simulink model "DynamicSimulator"  (R2016b)
settings: Solver=VariableStepAuto  StartTime=0.0  StopTime=inf  RelTol=1e-3
settings Model: Creator=Zikinkeria  LastModifiedBy=rcooper

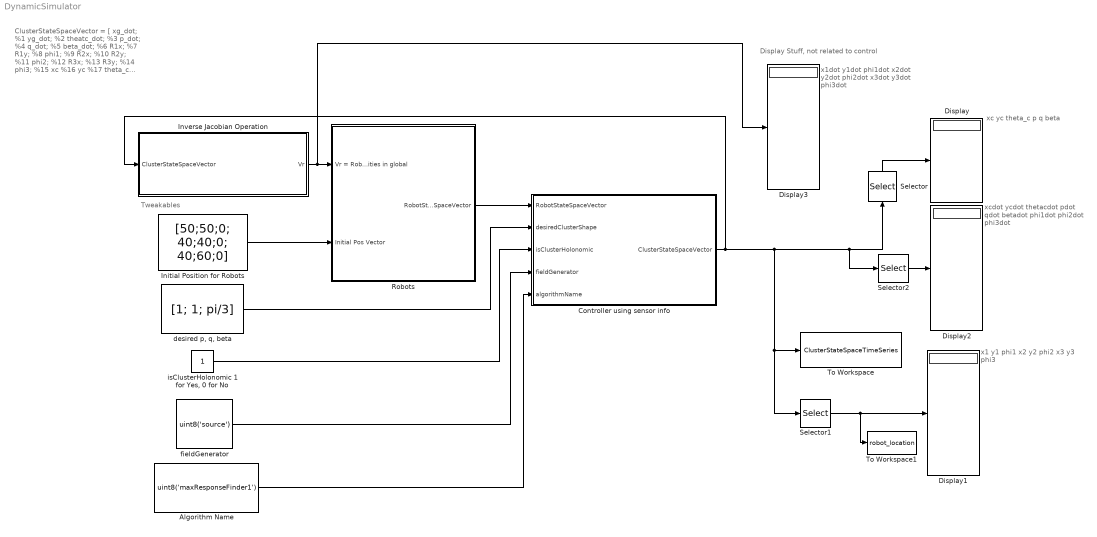
== system DynamicSimulator ==
  note: Tweakables
  note: Display Stuff, not related to control
  note: x1
      | y1
      | phi1
      | x2
      | y2
      | phi2
      | x3
      | y3
      | phi3
  note: xc
      | yc
      | theta_c
      | p
      | q
      | beta
  note: xcdot
      | ycdot
      | thetacdot
      | pdot
      | qdot
      | betadot
      | phi1dot
      | phi2dot
      | phi3dot
  note: x1dot
      | y1dot
      | phi1dot
      | x2dot
      | y2dot
      | phi2dot
      | x3dot
      | y3dot
      | phi3dot
  note: ClusterStateSpaceVector =
      | [
      |         xg_dot;         %1
      |         yg_dot;         %2
      |         theatc_dot;   %3
      |         p_dot;           %4
      |         q_dot;           %5
      |         beta_dot;      %6
      |         R1x;              %7
      |         R1y;              %8
      |         phi1;              %9
      |         R2x;              %10
      |         R2y;              %11
      |         phi2;              %12
      |         R3x;              %13
      |         R3y;              %14
      |         phi3;              %15
      |         xc                  %16
      |         yc                  %17
      |         theta_c          %18
      |         p                    %19
      |         q                    %20
      |         beta               %21
      |         phi1               %22
      |         phi2               %23
      |         phi3               %24
      |         xc_dot;          %25
      |         yc_dot;          %26
      |         ];
  Algorithm Name : Constant  Value=uint8('maxResponseFinder1')
  Controller using sensor info : Subsystem
  Display{,1..3} (4 alike) : Display
  Initial Position for Robots : Constant  Value=[50;50;0; 40;40;0; 40;60;0]  VectorParams1D=off
  Inverse Jacobian Operation : MATLAB Function  TreatAsAtomicUnit=on
  Robots : Subsystem
  Selector : Selector  InputPortWidth=26  IndexOptions=Index vector (dialog)  Indices=[16 17 18 19 20 21]  OutputSizes=1
  Selector1 : Selector  InputPortWidth=26  IndexOptions=Index vector (dialog)  Indices=[7, 8, 9, 10, 11, 12, 13, 14, 15]  OutputSizes=1
  Selector2 : Selector  InputPortWidth=26  IndexOptions=Index vector (dialog)  Indices=[25, 26, 3, 4, 5, 6, 22, 23, 24]  OutputSizes=1
  To Workspace : ToWorkspace  VariableName=ClusterStateSpaceTimeSeries  SaveFormat=Timeseries  SampleTime=-1
  To Workspace1 : ToWorkspace  VariableName=robot_location  SaveFormat=Timeseries  SampleTime=-1
  "desired p, q, beta" : Constant  Value=[1; 1; pi/3]
  fieldGenerator : Constant  Value=uint8('source')
  "isClusterHolonomic 1 for Yes, 0 for No" : Constant
  wires:
  Initial Position for Robots/1 -> Robots/2(Initial Pos Vector)
  Robots/1(RobotStateSpaceVector) -> Controller using sensor info/1(RobotStateSpaceVector)
  Controller using sensor info/1(ClusterStateSpaceVector) -> Inverse Jacobian Operation/1(ClusterStateSpaceVector), Selector/1, Selector2/1, Selector1/1, To Workspace/1
  Selector/1 -> Display/1
  Selector2/1 -> Display2/1
  Inverse Jacobian Operation/1(Vr) -> Robots/1(Vr = Robot Velocities in global), Display3/1
  Selector1/1 -> To Workspace1/1, Display1/1
  "desired p, q, beta"/1 -> Controller using sensor info/2(desiredClusterShape)
  "isClusterHolonomic 1 for Yes, 0 for No"/1 -> Controller using sensor info/3(isClusterHolonomic)
  fieldGenerator/1 -> Controller using sensor info/4(fieldGenerator)
  Algorithm Name/1 -> Controller using sensor info/5(algorithmName)

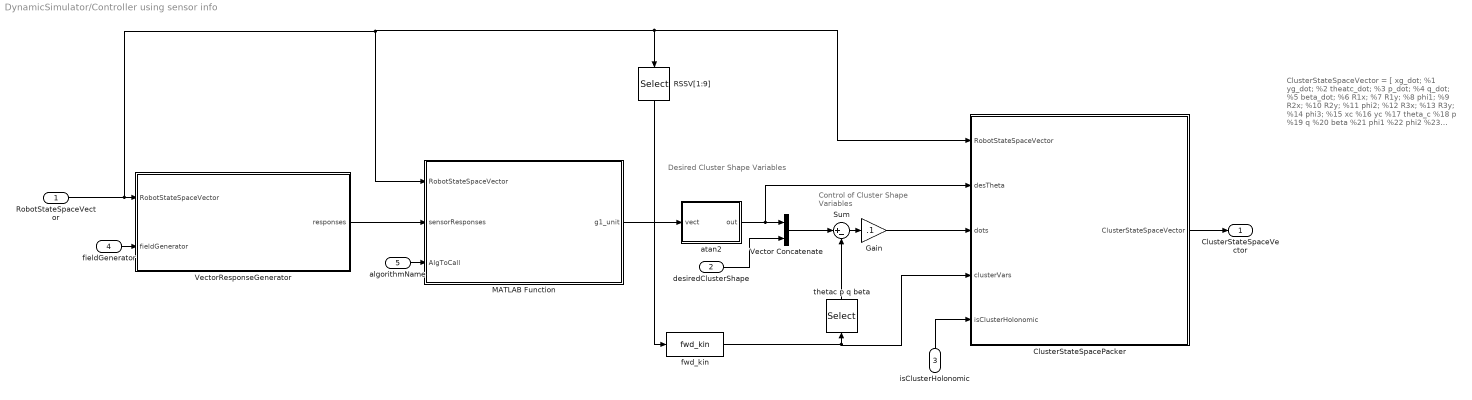
== system DynamicSimulator/Controller using sensor info ==
  note: Control of Cluster
      | Shape Variables
  note: Desired Cluster
      | Shape Variables
  note: ClusterStateSpaceVector = [
      |         xg_dot;         %1
      |         yg_dot;         %2
      |         theatc_dot;   %3
      |         p_dot;           %4
      |         q_dot;           %5
      |         beta_dot;      %6
      |         R1x;              %7
      |         R1y;              %8
      |         phi1;              %9
      |         R2x;              %10
      |         R2y;              %11
      |         phi2;              %12
      |         R3x;              %13
      |         R3y;              %14
      |         phi3;              %15
      |         xc                  %16
      |         yc                  %17
      |         theta_c          %18
      |         p                    %19
      |         q                    %20
      |         beta               %21
      |         phi1               %22
      |         phi2               %23
      |         phi3               %24
      |         xc_dot;          %25
      |         yc_dot;          %26
      |         ];
  RobotStateSpaceVector : Inport
  desiredClusterShape : Inport  Port=2
  isClusterHolonomic : Inport  Port=3
  fieldGenerator : Inport  Port=4
  algorithmName : Inport  Port=5
  ClusterStateSpacePacker : MATLAB Function  TreatAsAtomicUnit=on
  Gain : Gain  Gain=.1
  MATLAB Function : MATLAB Function  TreatAsAtomicUnit=on
  RSSV[1:9] : Selector  InputPortWidth=18  IndexOptions=Index vector (dialog)  Indices=[1 2 3 4 5 6 7 8 9]  OutputSizes=1
  Sum : Sum  Inputs=|+-
  Vector Concatenate : Concatenate
  VectorResponseGenerator : MATLAB Function  TreatAsAtomicUnit=on
  atan2 : MATLAB Function  TreatAsAtomicUnit=on
  fwd_kin : MATLABFcn  MATLABFcn=fwd_kin
  thetac p q beta : Selector  InputPortWidth=9  IndexOptions=Index vector (dialog)  Indices=[3 4 5 6]  OutputSizes=1
  ClusterStateSpaceVector : Outport
  wires:
  fieldGenerator/1 -> VectorResponseGenerator/2(fieldGenerator)
  algorithmName/1 -> MATLAB Function/3(AlgToCall)
  VectorResponseGenerator/1(responses) -> MATLAB Function/2(sensorResponses)
  RobotStateSpaceVector/1 -> MATLAB Function/1(RobotStateSpaceVector), ClusterStateSpacePacker/1(RobotStateSpaceVector), RSSV[1:9]/1, VectorResponseGenerator/1(RobotStateSpaceVector)
  RSSV[1:9]/1 -> fwd_kin/1
  fwd_kin/1 -> ClusterStateSpacePacker/4(clusterVars), thetac p q beta/1
  MATLAB Function/1(g1_unit) -> atan2/1(vect)
  atan2/1(out) -> ClusterStateSpacePacker/2(desTheta), Vector Concatenate/1
  desiredClusterShape/1 -> Vector Concatenate/2
  Vector Concatenate/1 -> Sum/1
  thetac p q beta/1 -> Sum/2
  ClusterStateSpacePacker/1(ClusterStateSpaceVector) -> ClusterStateSpaceVector/1
  isClusterHolonomic/1 -> ClusterStateSpacePacker/5(isClusterHolonomic)
  Sum/1 -> Gain/1
  Gain/1 -> ClusterStateSpacePacker/3(dots)

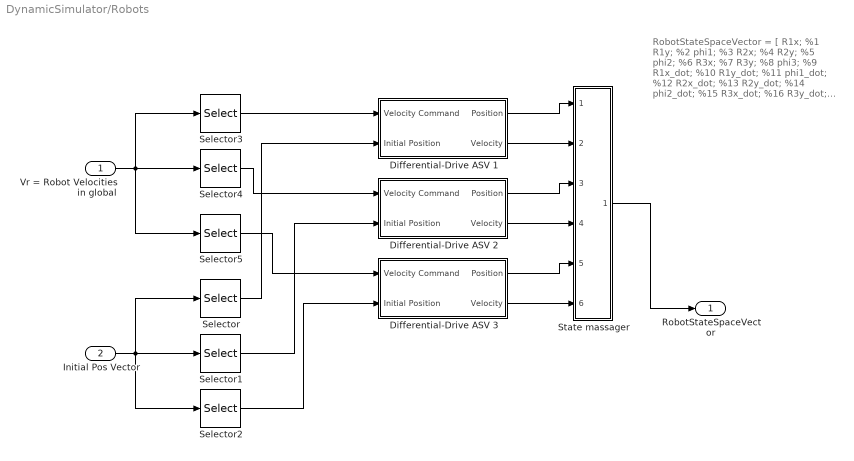
== system DynamicSimulator/Robots ==
  note: RobotStateSpaceVector =
      | [ R1x;        %1
      |   R1y;        %2
      |   phi1;        %3
      |   R2x;         %4
      |   R2y;         %5
      |   phi2;        %6
      |   R3x;         %7
      |   R3y;         %8
      |   phi3;         %9
      |   R1x_dot;  %10
      |   R1y_dot;  %11
      |   phi1_dot;  %12
      |   R2x_dot;  %13
      |   R2y_dot;  %14
      |   phi2_dot;  %15
      |   R3x_dot;  %16
      |   R3y_dot;  %17
      |   phi3_dot]; %18
      |
      |
      | all in the global frame
  Vr = Robot Velocities in global : Inport
  Initial Pos Vector : Inport  Port=2
  Differential-Drive ASV 1 : Subsystem
  Differential-Drive ASV 2 : Subsystem
  Differential-Drive ASV 3 : Subsystem
  Selector : Selector  InputPortWidth=9  IndexOptions=Index vector (dialog)  Indices=[1 2 3]  OutputSizes=1
  Selector1 : Selector  InputPortWidth=9  IndexOptions=Index vector (dialog)  Indices=[4 5 6]  OutputSizes=1
  Selector2 : Selector  InputPortWidth=9  IndexOptions=Index vector (dialog)  Indices=[7 8 9]  OutputSizes=1
  Selector3 : Selector  InputPortWidth=9  IndexOptions=Index vector (dialog)  Indices=[1 2 3]  OutputSizes=1
  Selector4 : Selector  InputPortWidth=9  IndexOptions=Index vector (dialog)  Indices=[4 5 6]  OutputSizes=1
  Selector5 : Selector  InputPortWidth=9  IndexOptions=Index vector (dialog)  Indices=[7 8 9]  OutputSizes=1
  State massager : Subsystem
  RobotStateSpaceVector : Outport
  wires:
  Selector4/1 -> Differential-Drive ASV 2/1(Velocity Command)
  Selector5/1 -> Differential-Drive ASV 3/1(Velocity Command)
  Selector2/1 -> Differential-Drive ASV 3/2(Initial Position)
  Selector1/1 -> Differential-Drive ASV 2/2(Initial Position)
  Initial Pos Vector/1 -> Selector/1, Selector2/1, Selector1/1
  Selector/1 -> Differential-Drive ASV 1/2(Initial Position)
  Differential-Drive ASV 1/1(Position) -> State massager/1(In1)
  Differential-Drive ASV 1/2(Velocity) -> State massager/2(In2)
  Differential-Drive ASV 2/1(Position) -> State massager/3(In3)
  Differential-Drive ASV 2/2(Velocity) -> State massager/4(In4)
  Differential-Drive ASV 3/1(Position) -> State massager/5(In5)
  Differential-Drive ASV 3/2(Velocity) -> State massager/6(In6)
  State massager/1(Out1) -> RobotStateSpaceVector/1
  Selector3/1 -> Differential-Drive ASV 1/1(Velocity Command)
  Vr = Robot Velocities in global/1 -> Selector3/1, Selector4/1, Selector5/1

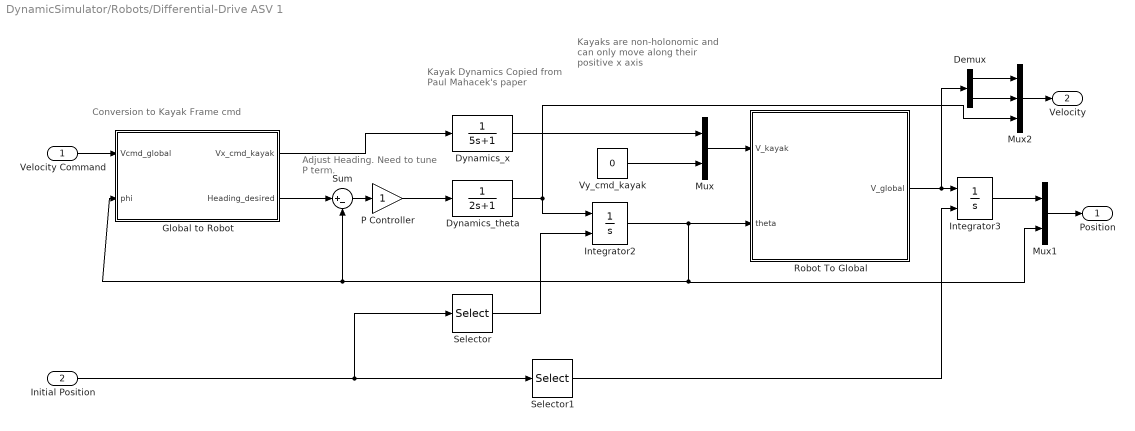
== system DynamicSimulator/Robots/Differential-Drive ASV 1 ==
  note: Conversion to Kayak Frame cmd
  note: Kayak Dynamics Copied from Paul Mahacek's paper
  note: Adjust Heading. Need to tune P term.
  note: Kayaks are non-holonomic and can only move along their positive x axis
  Velocity Command : Inport
  Initial Position : Inport  Port=2
  Demux : Demux  Outputs=2
  Dynamics_theta : TransferFcn  Denominator=[2 1]
  Dynamics_x : TransferFcn  Denominator=[5 1]
  Global to Robot : MATLAB Function  TreatAsAtomicUnit=on
  Integrator2 : Integrator  InitialConditionSource=external
  Integrator3 : Integrator  InitialConditionSource=external
  Mux : Mux  Inputs=2
  Mux1 : Mux  Inputs=2
  Mux2 : Mux  Inputs=3
  P Controller : Gain
  Robot To Global : MATLAB Function  TreatAsAtomicUnit=on
  Selector : Selector  InputPortWidth=3  IndexOptions=Index vector (dialog)  Indices=[3]  OutputSizes=1
  Selector1 : Selector  InputPortWidth=3  IndexOptions=Index vector (dialog)  Indices=[1 2]  OutputSizes=1
  Sum : Sum  Inputs=|+-
  Vy_cmd_kayak : Constant  Value=0
  Position : Outport
  Velocity : Outport  Port=2
  wires:
  Global to Robot/1(Vx_cmd_kayak) -> Dynamics_x/1
  Global to Robot/2(Heading_desired) -> Sum/1
  Sum/1 -> P Controller/1
  P Controller/1 -> Dynamics_theta/1
  Dynamics_theta/1 -> Mux2/3, Integrator2/1
  Initial Position/1 -> Selector1/1, Selector/1
  Mux/1 -> Robot To Global/1(V_kayak)
  Dynamics_x/1 -> Mux/1
  Vy_cmd_kayak/1 -> Mux/2
  Integrator2/1 -> Global to Robot/2(phi), Sum/2, Mux1/2, Robot To Global/2(theta)
  Robot To Global/1(V_global) -> Demux/1, Integrator3/1
  Selector/1 -> Integrator2/2
  Selector1/1 -> Integrator3/2
  Mux1/1 -> Position/1
  Integrator3/1 -> Mux1/1
  Demux/1 -> Mux2/1
  Demux/2 -> Mux2/2
  Mux2/1 -> Velocity/1
  Velocity Command/1 -> Global to Robot/1(Vcmd_global)

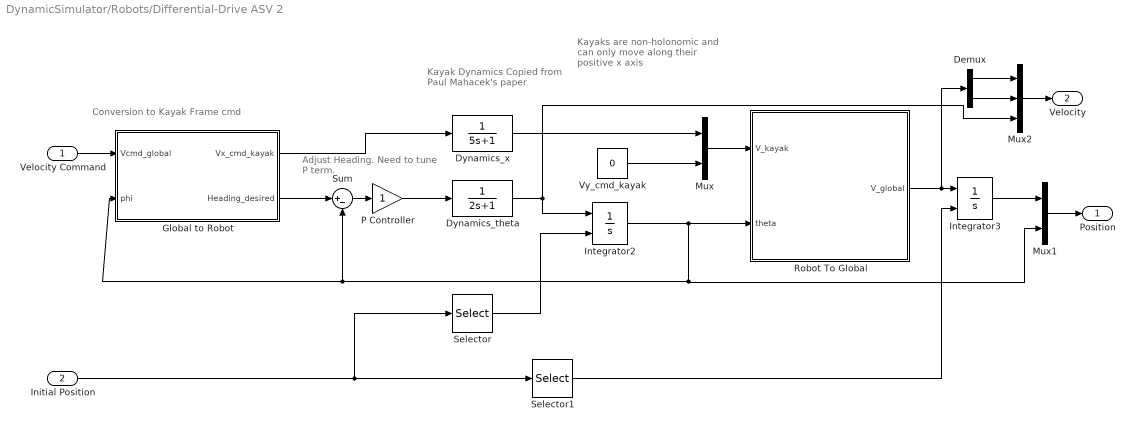
== system DynamicSimulator/Robots/Differential-Drive ASV 2 ==
  note: Conversion to Kayak Frame cmd
  note: Kayak Dynamics Copied from Paul Mahacek's paper
  note: Adjust Heading. Need to tune P term.
  note: Kayaks are non-holonomic and can only move along their positive x axis
  Velocity Command : Inport
  Initial Position : Inport  Port=2
  Demux : Demux  Outputs=2
  Dynamics_theta : TransferFcn  Denominator=[2 1]
  Dynamics_x : TransferFcn  Denominator=[5 1]
  Global to Robot : MATLAB Function  TreatAsAtomicUnit=on
  Integrator2 : Integrator  InitialConditionSource=external
  Integrator3 : Integrator  InitialConditionSource=external
  Mux : Mux  Inputs=2
  Mux1 : Mux  Inputs=2
  Mux2 : Mux  Inputs=3
  P Controller : Gain
  Robot To Global : MATLAB Function  TreatAsAtomicUnit=on
  Selector : Selector  InputPortWidth=3  IndexOptions=Index vector (dialog)  Indices=[3]  OutputSizes=1
  Selector1 : Selector  InputPortWidth=3  IndexOptions=Index vector (dialog)  Indices=[1 2]  OutputSizes=1
  Sum : Sum  Inputs=|+-
  Vy_cmd_kayak : Constant  Value=0
  Position : Outport
  Velocity : Outport  Port=2
  wires:
  Global to Robot/1(Vx_cmd_kayak) -> Dynamics_x/1
  Global to Robot/2(Heading_desired) -> Sum/1
  Sum/1 -> P Controller/1
  P Controller/1 -> Dynamics_theta/1
  Dynamics_theta/1 -> Mux2/3, Integrator2/1
  Initial Position/1 -> Selector1/1, Selector/1
  Mux/1 -> Robot To Global/1(V_kayak)
  Dynamics_x/1 -> Mux/1
  Vy_cmd_kayak/1 -> Mux/2
  Integrator2/1 -> Global to Robot/2(phi), Sum/2, Mux1/2, Robot To Global/2(theta)
  Robot To Global/1(V_global) -> Demux/1, Integrator3/1
  Selector/1 -> Integrator2/2
  Selector1/1 -> Integrator3/2
  Mux1/1 -> Position/1
  Integrator3/1 -> Mux1/1
  Demux/1 -> Mux2/1
  Demux/2 -> Mux2/2
  Mux2/1 -> Velocity/1
  Velocity Command/1 -> Global to Robot/1(Vcmd_global)

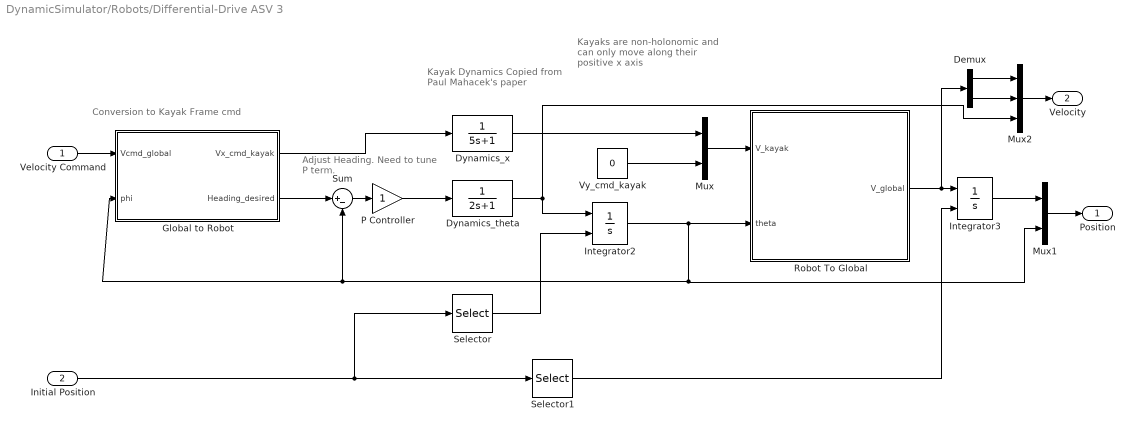
== system DynamicSimulator/Robots/Differential-Drive ASV 3 ==
  note: Conversion to Kayak Frame cmd
  note: Kayak Dynamics Copied from Paul Mahacek's paper
  note: Adjust Heading. Need to tune P term.
  note: Kayaks are non-holonomic and can only move along their positive x axis
  Velocity Command : Inport
  Initial Position : Inport  Port=2
  Demux : Demux  Outputs=2
  Dynamics_theta : TransferFcn  Denominator=[2 1]
  Dynamics_x : TransferFcn  Denominator=[5 1]
  Global to Robot : MATLAB Function  TreatAsAtomicUnit=on
  Integrator2 : Integrator  InitialConditionSource=external
  Integrator3 : Integrator  InitialConditionSource=external
  Mux : Mux  Inputs=2
  Mux1 : Mux  Inputs=2
  Mux2 : Mux  Inputs=3
  P Controller : Gain
  Robot To Global : MATLAB Function  TreatAsAtomicUnit=on
  Selector : Selector  InputPortWidth=3  IndexOptions=Index vector (dialog)  Indices=[3]  OutputSizes=1
  Selector1 : Selector  InputPortWidth=3  IndexOptions=Index vector (dialog)  Indices=[1 2]  OutputSizes=1
  Sum : Sum  Inputs=|+-
  Vy_cmd_kayak : Constant  Value=0
  Position : Outport
  Velocity : Outport  Port=2
  wires:
  Global to Robot/1(Vx_cmd_kayak) -> Dynamics_x/1
  Global to Robot/2(Heading_desired) -> Sum/1
  Sum/1 -> P Controller/1
  P Controller/1 -> Dynamics_theta/1
  Dynamics_theta/1 -> Mux2/3, Integrator2/1
  Initial Position/1 -> Selector1/1, Selector/1
  Mux/1 -> Robot To Global/1(V_kayak)
  Dynamics_x/1 -> Mux/1
  Vy_cmd_kayak/1 -> Mux/2
  Integrator2/1 -> Global to Robot/2(phi), Sum/2, Mux1/2, Robot To Global/2(theta)
  Robot To Global/1(V_global) -> Demux/1, Integrator3/1
  Selector/1 -> Integrator2/2
  Selector1/1 -> Integrator3/2
  Mux1/1 -> Position/1
  Integrator3/1 -> Mux1/1
  Demux/1 -> Mux2/1
  Demux/2 -> Mux2/2
  Mux2/1 -> Velocity/1
  Velocity Command/1 -> Global to Robot/1(Vcmd_global)

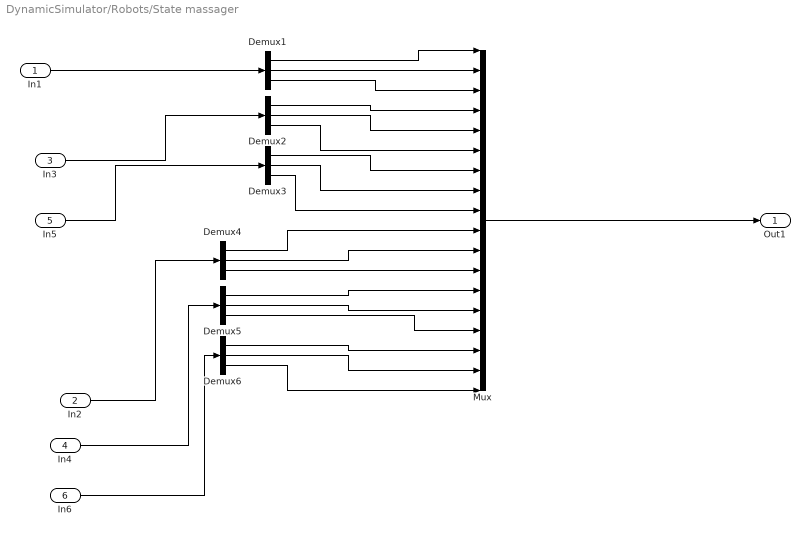
== system DynamicSimulator/Robots/State massager ==
  In1 : Inport
  In2 : Inport  Port=2
  In3 : Inport  Port=3
  In4 : Inport  Port=4
  In5 : Inport  Port=5
  In6 : Inport  Port=6
  Demux{1..6} (6 alike) : Demux  Outputs=3
  Mux : Mux  Inputs=18
  Out1 : Outport
  wires:
  Demux5/2 -> Mux/14
  Demux2/1 -> Mux/4
  Demux2/2 -> Mux/5
  Demux4/3 -> Mux/12
  Demux3/3 -> Mux/9
  Demux6/3 -> Mux/18
  Demux3/2 -> Mux/8
  Demux5/1 -> Mux/13
  Demux4/2 -> Mux/11
  Demux1/3 -> Mux/3
  Demux2/3 -> Mux/6
  Demux1/2 -> Mux/2
  Demux4/1 -> Mux/10
  Demux3/1 -> Mux/7
  Demux1/1 -> Mux/1
  Demux6/2 -> Mux/17
  Demux5/3 -> Mux/15
  Demux6/1 -> Mux/16
  In1/1 -> Demux1/1
  In4/1 -> Demux5/1
  In2/1 -> Demux4/1
  In3/1 -> Demux2/1
  In5/1 -> Demux3/1
  In6/1 -> Demux6/1
  Mux/1 -> Out1/1

== matlab function DynamicSimulator/Robots/Differential-Drive ASV 2/Global to Robot ==
  data: Vcmd_global input; Vx_cmd_kayak output; Heading_desired output; phi input
function [Vx_cmd_kayak,Heading_desired] = fcn(Vcmd_global, phi)
Vx_cmd_global = Vcmd_global(1);
Vy_cmd_global = Vcmd_global(2);

Heading_desired = atan2(Vy_cmd_global,Vx_cmd_global);
Vx_cmd_kayak = sqrt(Vx_cmd_global^2 + Vy_cmd_global^2)*cos(abs(Heading_desired-phi));

== matlab function DynamicSimulator/Robots/Differential-Drive ASV 2/Robot To Global ==
  data: V_kayak input; V_global output; theta input
function V_global = Robot_to_Frame_Transformation(V_kayak,theta)
%This function calculates the local robot velocities
%based on the global robot velocities

%Initialize Variables
V_robot = [V_kayak(1);V_kayak(2)];

T = [cos(theta) -sin(theta);...
    sin(theta) cos(theta)];
V_global = T*V_robot;

== matlab function DynamicSimulator/Robots/Differential-Drive ASV 3/Global to Robot ==
  data: Vcmd_global input; Vx_cmd_kayak output; Heading_desired output; phi input
function [Vx_cmd_kayak,Heading_desired] = fcn(Vcmd_global, phi)
Vx_cmd_global = Vcmd_global(1);
Vy_cmd_global = Vcmd_global(2);

Heading_desired = atan2(Vy_cmd_global,Vx_cmd_global);
Vx_cmd_kayak = sqrt(Vx_cmd_global^2 + Vy_cmd_global^2)*cos(abs(Heading_desired-phi));

== matlab function DynamicSimulator/Inverse Jacobian Operation ==
  data: ClusterStateSpaceVector input; Vr output
function Vr = inverse_jacobian( ClusterStateSpaceVector )
% This is for a three bot p,q,beta cluster, in aero frame
%ClusterStateSpaceVector = [
%         xg_dot;           %1
%         yg_dot;           %2
%         theatc_dot;       %3
%         p_dot;            %4
%         q_dot;            %5
%         beta_dot;         %6
%         R1x;              %7
%         R1y;              %8
%         phi1;             %9
%         R2x;              %10
%         R2y;              %11
%         phi2;             %12
%         R3x;              %13
%         R3y;              %14
%         phi3;             %15
%         xc                %16
%         yc                %17
%         theta_c           %18
%         p                 %19
%         q                 %20
%         beta              %21
%         phi1              %22
%         phi2              %23
%         phi3              %24
%         xc_dot;           %25
%         yc_dot;           %26
%         ];
theta_c = ClusterStateSpaceVector(18)
p = ClusterStateSpaceVector(19)
q = ClusterStateSpaceVector(20)
beta1 = ClusterStateSpaceVector(21)

inv_Jac = zeros(9, 9);
if nearBetaSingularity(beta1)
    inv_Jac = [1, 0, 0, 0, 0, 0, 0, 0, 0;
               0, 1, 0, 0, 0, 0, 0, 0, 0;
               0, 0, 1, 0, 0, 0, 1, 0, 0;
               1, 0, p*cos(theta_c), sin(theta_c), 0, 0, 0, 0, 0;
               0, 1, p*sin(theta_c), sin(theta_c), 0, 0, 0, 0, 0;
               0, 0, 1, 0, 0, 0, 0, 1, 0;
               1, 0, -q*cos(theta_c), 0, -sin(theta_c), 0, 0, 0, 0;
               0, 1, -q*sin(theta_c), 0, cos(theta_c), 0, 0, 0, 0;
               0, 0, 1, 0, 0, 0, 0, 0, 1];
else 
    inv_Jac = [ 1, 0, -(sin(theta_c)*(p^2 + 2*cos(beta1)*p*q + q^2)^(1/2))/3, (cos(theta_c)*(2*p + 2*q*cos(beta1)))/(6*(p^2 + 2*cos(beta1)*p*q + q^2)^(1/2)), (cos(theta_c)*(2*q + 2*p*cos(beta1)))/(6*(p^2 + 2*cos(beta1)*p*q + q^2)^(1/2)), -(p*q*sin(beta1)*cos(theta_c))/(3*(p^2 + 2*cos(beta1)*p*q + q^2)^(1/2)), 0, 0, 0;
        0, 1,  (cos(theta_c)*(p^2 + 2*cos(beta1)*p*q + q^2)^(1/2))/3, (sin(theta_c)*(2*p + 2*q*cos(beta1)))/(6*(p^2 + 2*cos(beta1)*p*q + q^2)^(1/2)), (sin(theta_c)*(2*q + 2*p*cos(beta1)))/(6*(p^2 + 2*cos(beta1)*p*q + q^2)^(1/2)), -(p*q*sin(beta1)*sin(theta_c))/(3*(p^2 + 2*cos(beta1)*p*q + q^2)^(1/2)), 0, 0, 0;
        0, 0, 1, 0, 0, 0, 1, 0, 0;
        1, 0, p*cos(theta_c)*(-(q^2*(cos(beta1)^2 - 1))/(p^2 + 2*cos(beta1)*p*q + q^2))^(1/2) + (sin(theta_c)*(2*p^2 + cos(beta1)*p*q - q^2))/(3*(p^2 + 2*cos(beta1)*p*q + q^2)^(1/2)),   sin(theta_c)*(-(q^2*(cos(beta1)^2 - 1))/(p^2 + 2*cos(beta1)*p*q + q^2))^(1/2) - (cos(theta_c)*(5*p*q^2 + 2*p^3 + 2*q^3*cos(beta1) + 6*p^2*q*cos(beta1) + p*q^2*cos(beta1)^2))/(3*(p^2 + 2*cos(beta1)*p*q + q^2)^(3/2)) + (p*q^2*sin(theta_c)*(p + q*cos(beta1))*(cos(beta1)^2 - 1))/((p^2 + 2*cos(beta1)*p*q + q^2)^2*(-(q^2*(cos(beta1)^2 - 1))/(p^2 + 2*cos(beta1)*p*q + q^2))^(1/2)), (cos(theta_c)*(4*p^2*q + q^3 + p^3*cos(beta1) + 3*p*q^2*cos(beta1) - p^2*q*cos(beta1)^2))/(3*(p^2 + 2*cos(beta1)*p*q + q^2)^(3/2)) - (p^2*q*sin(theta_c)*(p + q*cos(beta1))*(cos(beta1)^2 - 1))/((p^2 + 2*cos(beta1)*p*q + q^2)^2*(-(q^2*(cos(beta1)^2 - 1))/(p^2 + 2*cos(beta1)*p*q + q^2))^(1/2)), (p*q*sin(beta1)*cos(theta_c)*(- p^2 + cos(beta1)*p*q + 2*q^2))/(3*(p^2 + 2*cos(beta1)*p*q + q^2)^(3/2)) + (p*q^2*sin(beta1)*sin(theta_c)*(p^2*cos(beta1) + p*q*cos(beta1)^2 + p*q + q^2*cos(beta1)))/((p^2 + 2*cos(beta1)*p*q + q^2)^2*(-(q^2*(cos(beta1)^2 - 1))/(p^2 + 2*cos(beta1)*p*q + q^2))^(1/2)), 0, 0, 0;
        0, 1, p*sin(theta_c)*(-(q^2*(cos(beta1)^2 - 1))/(p^2 + 2*cos(beta1)*p*q + q^2))^(1/2) - (cos(theta_c)*(2*p^2 + cos(beta1)*p*q - q^2))/(3*(p^2 + 2*cos(beta1)*p*q + q^2)^(1/2)), - cos(theta_c)*(-(q^2*(cos(beta1)^2 - 1))/(p^2 + 2*cos(beta1)*p*q + q^2))^(1/2) - (sin(theta_c)*(5*p*q^2 + 2*p^3 + 2*q^3*cos(beta1) + 6*p^2*q*cos(beta1) + p*q^2*cos(beta1)^2))/(3*(p^2 + 2*cos(beta1)*p*q + q^2)^(3/2)) - (p*q^2*cos(theta_c)*(p + q*cos(beta1))*(cos(beta1)^2 - 1))/((p^2 + 2*cos(beta1)*p*q + q^2)^2*(-(q^2*(cos(beta1)^2 - 1))/(p^2 + 2*cos(beta1)*p*q + q^2))^(1/2)), (sin(theta_c)*(4*p^2*q + q^3 + p^3*cos(beta1) + 3*p*q^2*cos(beta1) - p^2*q*cos(beta1)^2))/(3*(p^2 + 2*cos(beta1)*p*q + q^2)^(3/2)) + (p^2*q*cos(theta_c)*(p + q*cos(beta1))*(cos(beta1)^2 - 1))/((p^2 + 2*cos(beta1)*p*q + q^2)^2*(-(q^2*(cos(beta1)^2 - 1))/(p^2 + 2*cos(beta1)*p*q + q^2))^(1/2)), (p*q*sin(beta1)*sin(theta_c)*(- p^2 + cos(beta1)*p*q + 2*q^2))/(3*(p^2 + 2*cos(beta1)*p*q + q^2)^(3/2)) - (p*q^2*sin(beta1)*cos(theta_c)*(p^2*cos(beta1) + p*q*cos(beta1)^2 + p*q + q^2*cos(beta1)))/((p^2 + 2*cos(beta1)*p*q + q^2)^2*(-(q^2*(cos(beta1)^2 - 1))/(p^2 + 2*cos(beta1)*p*q + q^2))^(1/2)), 0, 0, 0;
        0, 0, 1, 0, 0, 0, 0, 1, 0;
        1, 0, (sin(theta_c)*(- p^2 + cos(beta1)*p*q + 2*q^2))/(3*(p^2 + 2*cos(beta1)*p*q + q^2)^(1/2)) - q*cos(theta_c)*(-(p^2*(cos(beta1)^2 - 1))/(p^2 + 2*cos(beta1)*p*q + q^2))^(1/2),                                                                                       (cos(theta_c)*(4*p*q^2 + p^3 + q^3*cos(beta1) + 3*p^2*q*cos(beta1) - p*q^2*cos(beta1)^2))/(3*(p^2 + 2*cos(beta1)*p*q + q^2)^(3/2)) + (p*q^2*sin(theta_c)*(q + p*cos(beta1))*(cos(beta1)^2 - 1))/((p^2 + 2*cos(beta1)*p*q + q^2)^2*(-(p^2*(cos(beta1)^2 - 1))/(p^2 + 2*cos(beta1)*p*q + q^2))^(1/2)), - sin(theta_c)*(-(p^2*(cos(beta1)^2 - 1))/(p^2 + 2*cos(beta1)*p*q + q^2))^(1/2) - (cos(theta_c)*(5*p^2*q + 2*q^3 + 2*p^3*cos(beta1) + 6*p*q^2*cos(beta1) + p^2*q*cos(beta1)^2))/(3*(p^2 + 2*cos(beta1)*p*q + q^2)^(3/2)) - (p^2*q*sin(theta_c)*(q + p*cos(beta1))*(cos(beta1)^2 - 1))/((p^2 + 2*cos(beta1)*p*q + q^2)^2*(-(p^2*(cos(beta1)^2 - 1))/(p^2 + 2*cos(beta1)*p*q + q^2))^(1/2)),   (p*q*sin(beta1)*cos(theta_c)*(2*p^2 + cos(beta1)*p*q - q^2))/(3*(p^2 + 2*cos(beta1)*p*q + q^2)^(3/2)) - (p^2*q*sin(beta1)*sin(theta_c)*(p^2*cos(beta1) + p*q*cos(beta1)^2 + p*q + q^2*cos(beta1)))/((p^2 + 2*cos(beta1)*p*q + q^2)^2*(-(p^2*(cos(beta1)^2 - 1))/(p^2 + 2*cos(beta1)*p*q + q^2))^(1/2)), 0, 0, 0;
        0, 1, - q*sin(theta_c)*(-(p^2*(cos(beta1)^2 - 1))/(p^2 + 2*cos(beta1)*p*q + q^2))^(1/2) - (cos(theta_c)*(- p^2 + cos(beta1)*p*q + 2*q^2))/(3*(p^2 + 2*cos(beta1)*p*q + q^2)^(1/2)), (sin(theta_c)*(4*p*q^2 + p^3 + q^3*cos(beta1) + 3*p^2*q*cos(beta1) - p*q^2*cos(beta1)^2))/(3*(p^2 + 2*cos(beta1)*p*q + q^2)^(3/2)) - (p*q^2*cos(theta_c)*(q + p*cos(beta1))*(cos(beta1)^2 - 1))/((p^2 + 2*cos(beta1)*p*q + q^2)^2*(-(p^2*(cos(beta1)^2 - 1))/(p^2 + 2*cos(beta1)*p*q + q^2))^(1/2)),   cos(theta_c)*(-(p^2*(cos(beta1)^2 - 1))/(p^2 + 2*cos(beta1)*p*q + q^2))^(1/2) - (sin(theta_c)*(5*p^2*q + 2*q^3 + 2*p^3*cos(beta1) + 6*p*q^2*cos(beta1) + p^2*q*cos(beta1)^2))/(3*(p^2 + 2*cos(beta1)*p*q + q^2)^(3/2)) + (p^2*q*cos(theta_c)*(q + p*cos(beta1))*(cos(beta1)^2 - 1))/((p^2 + 2*cos(beta1)*p*q + q^2)^2*(-(p^2*(cos(beta1)^2 - 1))/(p^2 + 2*cos(beta1)*p*q + q^2))^(1/2)),   (p*q*sin(beta1)*sin(theta_c)*(2*p^2 + cos(beta1)*p*q - q^2))/(3*(p^2 + 2*cos(beta1)*p*q + q^2)^(3/2)) + (p^2*q*sin(beta1)*cos(theta_c)*(p^2*cos(beta1) + p*q*cos(beta1)^2 + p*q + q^2*cos(beta1)))/((p^2 + 2*cos(beta1)*p*q + q^2)^2*(-(p^2*(cos(beta1)^2 - 1))/(p^2 + 2*cos(beta1)*p*q + q^2))^(1/2)), 0, 0, 0;
        0, 0, 1, 0, 0, 0, 0, 0, 1];
end
Vc = [ ClusterStateSpaceVector(25); % xc_dot        %1
       ClusterStateSpaceVector(26); % yc_dot        %2
       ClusterStateSpaceVector(3);  % thetac_dot    %3
       ClusterStateSpaceVector(4);  % p_dot         %4
       ClusterStateSpaceVector(5);  % q_dot         %5
       ClusterStateSpaceVector(6);  % beta_dot      %6
       ClusterStateSpaceVector(22); % phi1_dot      %7
       ClusterStateSpaceVector(23); % phi2_dot      %8
       ClusterStateSpaceVector(24)];% phi3_dot      %9

Vr = inv_Jac*Vc;
end

== matlab function DynamicSimulator/Robots/Differential-Drive ASV 1/Global to Robot ==
  data: Vcmd_global input; Vx_cmd_kayak output; Heading_desired output; phi input
function [Vx_cmd_kayak,Heading_desired] = fcn(Vcmd_global, phi)
Vx_cmd_global = Vcmd_global(1);
Vy_cmd_global = Vcmd_global(2);

Heading_desired = atan2(Vy_cmd_global,Vx_cmd_global);
Vx_cmd_kayak = sqrt(Vx_cmd_global^2 + Vy_cmd_global^2)*cos(abs(Heading_desired-phi));

== matlab function DynamicSimulator/Robots/Differential-Drive ASV 1/Robot To Global ==
  data: V_kayak input; V_global output; theta input
function V_global = Robot_to_Frame_Transformation(V_kayak,theta)
%This function calculates the local robot velocities
%based on the global robot velocities

%Initialize Variables
V_robot = [V_kayak(1);V_kayak(2)];

T = [cos(theta) -sin(theta);...
    sin(theta) cos(theta)];
V_global = T*V_robot;

== matlab function DynamicSimulator/Robots/Differential-Drive ASV 3/Robot To Global ==
  data: V_kayak input; V_global output; theta input
function V_global = Robot_to_Frame_Transformation(V_kayak,theta)
%This function calculates the local robot velocities
%based on the global robot velocities

%Initialize Variables
V_robot = [V_kayak(1);V_kayak(2)];

T = [cos(theta) -sin(theta);...
    sin(theta) cos(theta)];
V_global = T*V_robot;

== matlab function DynamicSimulator/Controller using sensor info/atan2 ==
  data: vect input; out output
function out = atan2_block(vect)
    out = atan2(vect(2), vect(1));
end

== matlab function DynamicSimulator/Controller using sensor info/MATLAB Function ==
  data: RobotStateSpaceVector input; g1_unit output; sensorResponses input; AlgToCall input
function g1_unit = AlgorithmCaller(RobotStateSpaceVector, sensorResponses, AlgToCall)
% This function feeds the RobotStateSpaceVector to the algorithm that uses
% the vector field sensorResponses to determine the "gradients" response.
%RobotStateSpaceVector = [ 
%    R1x;       %1
%    R1y;       %2
%    phi1;      %3
%    R2x;       %4
%    R2y;       %5
%    phi2;      %6
%    R3x;       %7
%    R3y;       %8
%    phi3;      %9
%    R1x_dot;   %10
%    R1y_dot;   %11
%    phi1_dot;  %12
%    R2x_dot;   %13
%    R2y_dot;   %14
%    phi2_dot;  %15
%    R3x_dot;   %16
%    R3y_dot;   %17
%    phi3_dot]; %18
    AlgToCall = char(AlgToCall);
    g1_unit = zeros(3, 1);
    g1_unit = feval(AlgToCall, RobotStateSpaceVector(1:3), RobotStateSpaceVector(4:6), RobotStateSpaceVector(7:9), sensorResponses);
end

== matlab function DynamicSimulator/Controller using sensor info/ClusterStateSpacePacker ==
  data: RobotStateSpaceVector input; desTheta input; dots input; clusterVars input; ClusterStateSpaceVector output; isClusterHolonomic input
function ClusterStateSpaceVector = ClusterStateSpacePacker(RobotStateSpaceVector, desTheta, dots, clusterVars, isClusterHolonomic)
%RobotStateSpaceVector = [ 
%    R1x;       %1
%    R1y;       %2
%    phi1;      %3
%    R2x;       %4
%    R2y;       %5
%    phi2;      %6
%    R3x;       %7
%    R3y;       %8
%    phi3;      %9
%    R1x_dot;   %10
%    R1y_dot;   %11
%    phi1_dot;  %12
%    R2x_dot;   %13
%    R2y_dot;   %14
%    phi2_dot;  %15
%    R3x_dot;   %16
%    R3y_dot;   %17
%    phi3_dot]; %18    
    if isClusterHolonomic
       yc_dot = sin(desTheta);
       xc_dot = cos(desTheta);
    else
       yc_dot = 0;
       xc_dot = 1; % makes the command non holonomic
    end

    Rgc = [cos(clusterVars(3)), -sin(clusterVars(3));
            sin(clusterVars(3)), cos(clusterVars(3))];
       
    %Transformation into global frame
    vg_dot = Rgc*([xc_dot yc_dot]');
    xg_dot = vg_dot(1);
    yg_dot = vg_dot(2);
    
    
    %The following command is just a test to make sure everything else is working
    %by sending cluster velocity command to the same way we did for cluster
    %position control.
    %{
    gain = 0.1;
    xc_dot = (50 - clusterVars(1))*gain;
    yc_dot = (25 - clusterVars(2))*gain;
    thetac_dot = (pi/2 - clusterVars(3))*gain;
    p_dot = (2 - clusterVars(4))*gain;
    q_dot = (2 - clusterVars(5))*gain;
    beta_dot = (pi/2 - clusterVars(6))*gain;
    
    %}
    
    ClusterStateSpaceVector = zeros(26,1);
    ClusterStateSpaceVector = [
        xg_dot;                                 %1
        yg_dot;                                 %2
        dots(1);                    %thetac_dot %3
        dots(2);                    %p_dot      %4
        dots(3);                    %q_dot      %5
        dots(4);                    %beta_dot   %6
        RobotStateSpaceVector(1);   %R1x        %7
        RobotStateSpaceVector(2);   %R1y        %8
        RobotStateSpaceVector(3);   %phi1       %9
        RobotStateSpaceVector(4);   %R2x        %10
        RobotStateSpaceVector(5);   %R2y        %11
        RobotStateSpaceVector(6);   %phi2       %12
        RobotStateSpaceVector(7);   %R3x        %13
        RobotStateSpaceVector(8);   %R3y        %14
        RobotStateSpaceVector(9);   %phi3       %15
        clusterVars(1);             %xc         %16
        clusterVars(2);             %yc         %17
        clusterVars(3);             %theta_c    %18
        clusterVars(4);             %p          %19
        clusterVars(5);             %q          %20
        clusterVars(6);             %beta       %21
        RobotStateSpaceVector(12);  %phi1_dot   %22
        RobotStateSpaceVector(15);  %phi2_dot   %23
        RobotStateSpaceVector(18);  %phi3_dot   %24
        xc_dot;                                 %25
        yc_dot;                                 %26
        ];
end

== matlab function DynamicSimulator/Controller using sensor info/VectorResponseGenerator ==
  data: RobotStateSpaceVector input; responses output size=[3,2]; fieldGenerator input
function responses = VectorResponseGenerator(RobotStateSpaceVector, fieldGenerator)
    %RobotStateSpaceVector = [ 
    %    R1x;       %1
    %    R1y;       %2
    %    phi1;      %3
    %    R2x;       %4
    %    R2y;       %5
    %    phi2;      %6
    %    R3x;       %7
    %    R3y;       %8
    %    phi3;      %9
    %    R1x_dot;   %10
    %    R1y_dot;   %11
    %    phi1_dot;  %12
    %    R2x_dot;   %13
    %    R2y_dot;   %14
    %    phi2_dot;  %15
    %    R3x_dot;   %16
    %    R3y_dot;   %17
    %    phi3_dot]; %18
    fieldGenerator = char(fieldGenerator);
    R1 = feval(fieldGenerator, RobotStateSpaceVector(1), RobotStateSpaceVector(2));
    R2 = feval(fieldGenerator, RobotStateSpaceVector(4), RobotStateSpaceVector(5));
    R3 = feval(fieldGenerator, RobotStateSpaceVector(7), RobotStateSpaceVector(8));
    responses = zeros(3,2);
    responses = [R1; R2; R3];
end
